simulink model "threetank_PS"  (Simulink 6.5)
settings: Solver=FixedStepDiscrete  StartTime=0.0  StopTime=200  FixedStep=0.03  RelTol=1e-3
values from neighbouring files (symbols this model uses):
  G = 0    [Threetank.m]
  H = vs1*sysd.c*sysd.b    [Threetank.m]    (also in data_with_uncertianty_generation.m = waitbar(0,'Please wait.','CreateCancelBtn',@btnWaitbarCancel; fault_data_generation.m = waitbar(0,'Please wait.','CreateCancelBtn',@btnWaitbarCancel)
  Hus = [Hus;help]    [Threetank.m]
  L = -vs0    [Threetank.m]
  Q = [0,0]    [Threetank.m]    (also in threetank.m = [Q1 Q2]')
  sysd = c2d(sys,0.03,'zoh')    [Threetank.m]
  V = vs1    [Threetank.m]
  vs = [1 2 3]*N    [Threetank.m]
  W = 1    [Threetank.m]
libraries: simulink x2
settings Model: Creator=AKS USER  LastModifiedBy=AKS USER
settings DebuggingCC: MultiTaskDSMMsg=warning  MultiTaskCondExecSysMsg=none
settings RTWCC: IncludeERTFirstTime=on

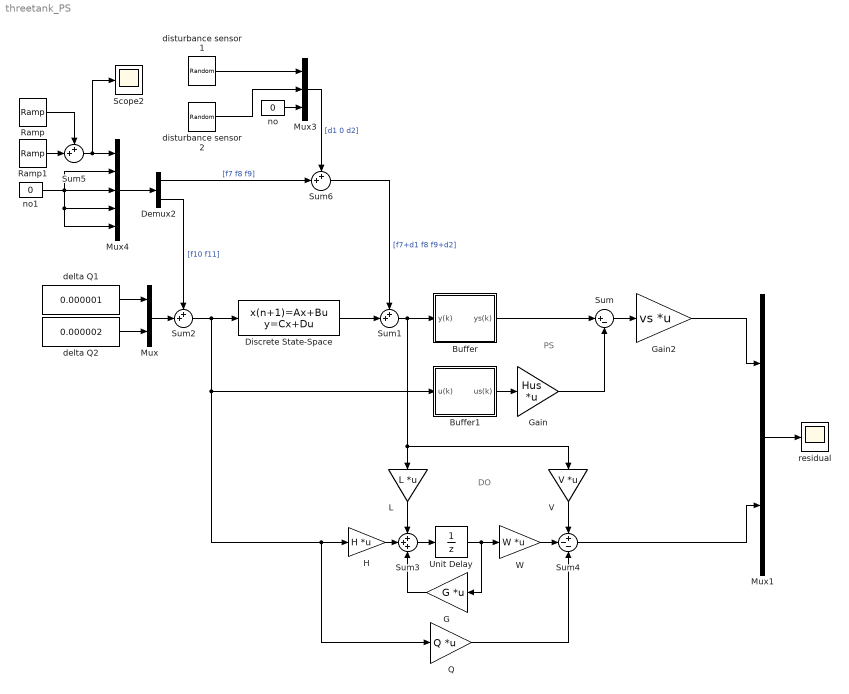
== system threetank_PS ==
  note: DO
  note: PS
  Buffer : Subsystem
  Buffer1 : Subsystem
  Demux2 : Demux  Outputs=2
  Discrete State-Space : DiscreteStateSpace  A=sysd.A  B=sysd.B  C=sysd.C  D=sysd.D  X0=[0,0,0]  SampleTime=-1
  G : Gain  Orientation=left  Gain=G  Multiplication=Matrix(K*u)
  Gain : Gain  Gain=Hus  Multiplication=Matrix(K*u)
  Gain2 : Gain  Gain=vs  Multiplication=Matrix(K*u)
  H : Gain  Gain=H  Multiplication=Matrix(K*u)
  L : Gain  Orientation=down  Gain=L  Multiplication=Matrix(K*u)
  Mux : Mux  Inputs=2
  Mux1 : Mux  Inputs=2
  Mux3 : Mux  Inputs=3
  Mux4 : Mux  Inputs=5
  Q : Gain  Gain=Q  Multiplication=Matrix(K*u)
  Ramp : simulink/Sources/Ramp  SystemSampleTime=-1  slope=0.001  start=50  X0=0
  Ramp1 : simulink/Sources/Ramp  SystemSampleTime=-1  slope=-0.001  start=80  X0=0
  Scope2 : Scope
      settings: TimeRange=999.99  SaveName=ScopeData2
  Sum : Sum  Inputs=|+-
  Sum{1..2,5..6} (4 alike) : Sum  Inputs=++|
  Sum3 : Sum  Inputs=+++
  Sum4 : Sum  Inputs=+--
  Unit Delay : UnitDelay  SampleTime=-1
  V : Gain  Orientation=down  Gain=V  Multiplication=Matrix(K*u)
  W : Gain  Gain=W  Multiplication=Matrix(K*u)
  delta Q1 : Constant  Value=0.000001  OutDataType=sfix(16)  ConRadixGroup=Use specified scaling  OutScaling=2^0  SampleTime=inf  FramePeriod=inf
  delta Q2 : Constant  Value=0.000002  OutDataType=sfix(16)  ConRadixGroup=Use specified scaling  OutScaling=2^0  SampleTime=inf  FramePeriod=inf
  disturbance sensor 1 : UniformRandomNumber  Minimum=-0.000001  Maximum=0.000001  SampleTime=0.03
  disturbance sensor 2 : UniformRandomNumber  Minimum=-0.000001  Maximum=0.000001  SampleTime=0.03
  no : Constant  Value=0  OutDataType=sfix(16)  ConRadixGroup=Use specified scaling  OutScaling=2^0  SampleTime=inf  FramePeriod=inf
  no1 : Constant  Value=0  OutDataType=sfix(16)  ConRadixGroup=Use specified scaling  OutScaling=2^0  SampleTime=inf  FramePeriod=inf
  residual : Scope
      settings: TimeRange=999.99
  wires:
  delta Q2/1 -> Mux/2
  delta Q1/1 -> Mux/1
  Buffer1/1(us(k)) -> Gain/1
  Gain/1 -> Sum/2
  Buffer/1(ys(k)) -> Sum/1
  Sum/1 -> Gain2/1
  Discrete State-Space/1 -> Sum1/2
  Sum1/1 -> Buffer/1(y(k)), V/1, L/1
  Gain2/1 -> Mux1/1
  Ramp/1 -> Sum5/1
  Ramp1/1 -> Sum5/2
  disturbance sensor 1/1 -> Mux3/1
  Demux2/2 -> Sum2/1  "[f10 f11]"
  Demux2/1 -> Sum6/2  "[f7 f8 f9]"
  Sum6/1 -> Sum1/1  "[f7+d1 f8 f9+d2]"
  disturbance sensor 2/1 -> Mux3/2
  no/1 -> Mux3/3
  Mux3/1 -> Sum6/1  "[d1 0 d2]"
  Sum5/1 -> Scope2/1, Mux4/1
  Mux4/1 -> Demux2/1
  no1/1 -> Mux4/3, Mux4/2, Mux4/4, Mux4/5
  Mux/1 -> Sum2/2
  Sum2/1 -> Discrete State-Space/1, Buffer1/1(u(k)), H/1, Q/1
  Unit Delay/1 -> G/1, W/1
  Sum3/1 -> Unit Delay/1
  H/1 -> Sum3/2
  G/1 -> Sum3/3
  L/1 -> Sum3/1
  V/1 -> Sum4/1
  W/1 -> Sum4/2
  Sum4/1 -> Mux1/2
  Mux1/1 -> residual/1
  Q/1 -> Sum4/3

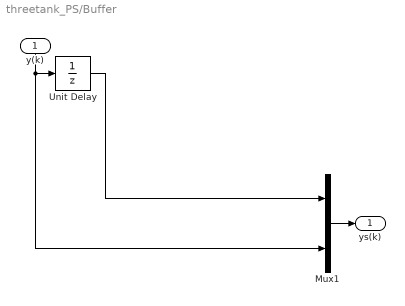
== system threetank_PS/Buffer ==
  y(k) : Inport  Orientation=down
  Mux1 : Mux  Inputs=2
  Unit Delay : UnitDelay  SampleTime=-1
  ys(k) : Outport
  wires:
  Mux1/1 -> ys(k)/1
  y(k)/1 -> Mux1/2, Unit Delay/1
  Unit Delay/1 -> Mux1/1

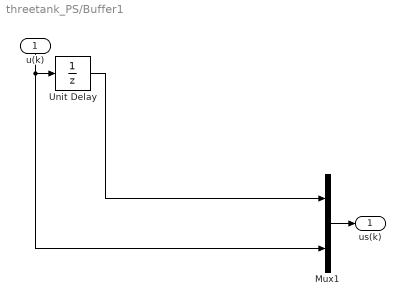
== system threetank_PS/Buffer1 ==
  u(k) : Inport  Orientation=down
  Mux1 : Mux  Inputs=2
  Unit Delay : UnitDelay  SampleTime=-1
  us(k) : Outport
  wires:
  Unit Delay/1 -> Mux1/1
  u(k)/1 -> Unit Delay/1, Mux1/2
  Mux1/1 -> us(k)/1
